simulink library "PlanarVehicle"  (R2018b)
settings: Solver=VariableStepAuto  StartTime=0.0  StopTime=10.0  RelTol=1e-3
undefined symbols (not defined in the file or in its folder): ENVIRONMENT, GEOMETRY, PROPULSION, SIMULATION
libraries: UWSimulink3DAnimationBlockset x2, UWAerospaceBlockset_FlightParameters x2, vrlib x1, UWMiscBlockset x1
settings Model: Creator=Christopher  LastModifiedBy=Christopher

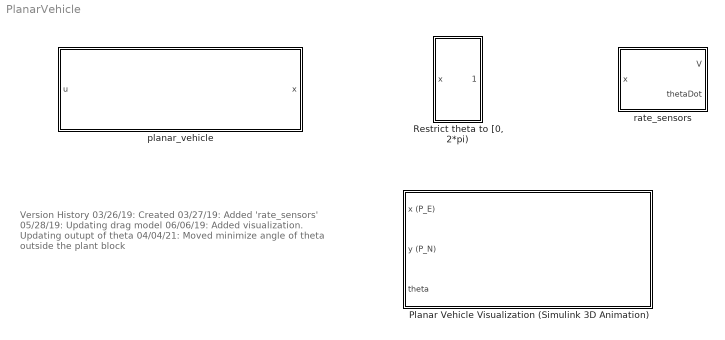
== system PlanarVehicle ==
  note: Version History
      | 03/26/19: Created
      | 03/27/19: Added 'rate_sensors'
      | 05/28/19: Updating drag model
      | 06/06/19: Added visualization.  Updating outupt of theta
      | 04/04/21: Moved minimize angle of theta outside the plant block
  Planar Vehicle Visualization (Simulink 3D Animation) : Subsystem  mask{T_animate=1}
      mask prompts: T_animate "Time step for animation"
      mask help:
      | This is a visualization of the planar vehicle using the Simulink 3D Animation environment.
      |
      | Note: Simulink should open up the VRML sink and it should display the aircraft model in a separate window.  If this does not occur, you may need to look under the mask and through down through subsystems until you find the VR Sink block.  Double click on this block to open the animation window.
      |
      | Further note that Simulink may close the VRML sink the first time it is run (it may display a warning with verbiage about 'Virtual world has been closed from outside of Simulink.'.  If this occurs, simply repeat the procedure of looking under the mask and double clicking on the VR Sink.
      |
      | INPUTS:
      | -x: x-position (position east)
      | -y: y-position (position north)
      | -theta: heading angle (0 = pointing in +y (east) direction, positive counter-clockwise) (rad)
      |
      | Christopher Lum
      | lum@uw.edu
      mask Display: image('Simulink3Visualization.png')
  "Restrict theta to [0, 2*pi)" : Subsystem
  planar_vehicle : Subsystem  mask{m=GEOMETRY.mass, Ib=GEOMETRY.Ib, Fmax=PROPULSION.Fmax, Mmax=PROPULSION.Mmax, x0=SIMULATION.X_0, CT=ENVIRONMENT.CT, CR=ENVIRONMENT.CR}
      mask prompts: m "Mass (kg)"; Ib "Moment of Inertia (kg*m^2)"; Fmax "Maximum thrust (N)"; Mmax "Maximum torque (N*m)"; x0 "Initial condition (6x1 vector)"; CT "Coefficient of translational friction (N*s^2/m^2)"; CR "Coefficient of rotational friction (N*m*s)"
      mask help:
      | Represent a simple planar model.
      |
      | The state vector is
      |
      |    x =  [x;y;xdot;ydot;theta;thetadot]
      |
      | The control vector is
      |
      |    u = [u1; u2]
      |
      | where:
      | u1 = fraction of  axial thrust force in range [-1, 1] (-1 = full nagative force, +1 = full positive force)
      | u2 = fraction of moment about CG in range [-1, 1] (-1 = full negative moment, +1 = full positive moment)
      |
      | INPUTS:
      | -u: 2x1 control vector
      |
      | OUTPUTS:
      | -x: 6x1 state vector
      |
      | For more information see PlanarVehicle.nb.
      |
      | Created by Christopher Lum
      | lum@uw.edu
      mask DialogControl Container5 Prompt: Geometry
      mask DialogControl Container9 Prompt: Propulsion
      mask DialogControl Container11 Prompt: Simulation
      mask DialogControl Container15 Prompt: Environment
      mask Display: image('Boat.png')
  rate_sensors : Subsystem
      mask help:
      | Models rate sensors which measure the translational and rotational velocity of the vehicle.
      |
      | INPUTS:
      | -x: 6x1 state vector
      |
      | OUTPUTS:
      | -V: scalar representing planar velocity (m/s)
      | -thetaDot: scalar representing rotational velocity (rad/s)
      |
      | Created by Christopher Lum
      | lum@uw.edu

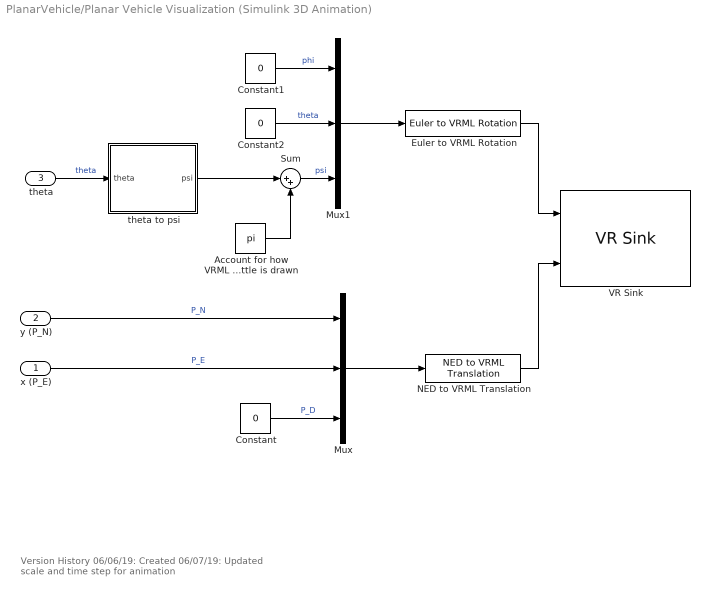
== system PlanarVehicle/Planar Vehicle Visualization (Simulink 3D Animation) ==
  note: Version History
      | 06/06/19: Created
      | 06/07/19: Updated scale and time step for animation
  x (P_E) : Inport
  y (P_N) : Inport  Port=2
  theta : Inport  Port=3
  Account for how VRML Shuttle is drawn : Constant  Value=pi
  Constant : Constant  Value=0
  Constant1 : Constant  Value=0
  Constant2 : Constant  Value=0
  Euler to VRML Rotation : UWSimulink3DAnimationBlockset/Euler to VRML Rotation
  Mux : Mux  Inputs=3
  Mux1 : Mux  Inputs=3
  NED to VRML Translation : UWSimulink3DAnimationBlockset/NED to VRML Translation
  Sum : Sum  Inputs=|++
  VR Sink : vrlib/VR Sink  InstantiateOnLoad=on  SampleTime=T_animate  ViewEnable=on  RemoteChange=off  RemoteView=off  FieldsWritten=Shuttle.rotation.4.1.1.double#Shuttle.translation.3.1.1.double  WorldFileName=PugetSound.wrl  AutoView=on  VideoDimensions=[]  AllowVariableSize=off
      settings: SourceProductBaseCode=VR
  theta to psi : Subsystem
  wires:
  Euler to VRML Rotation/1 -> VR Sink/1
  y (P_N)/1 -> Mux/1  "P_N"
  theta/1 -> theta to psi/1(theta)  "theta"
  Sum/1 -> Mux1/3  "psi"
  Constant2/1 -> Mux1/2  "theta"
  Account for how VRML Shuttle is drawn/1 -> Sum/2
  theta to psi/1(psi) -> Sum/1
  x (P_E)/1 -> Mux/2  "P_E"
  NED to VRML Translation/1 -> VR Sink/2
  Mux1/1 -> Euler to VRML Rotation/1
  Mux/1 -> NED to VRML Translation/1
  Constant/1 -> Mux/3  "P_D"
  Constant1/1 -> Mux1/1  "phi"

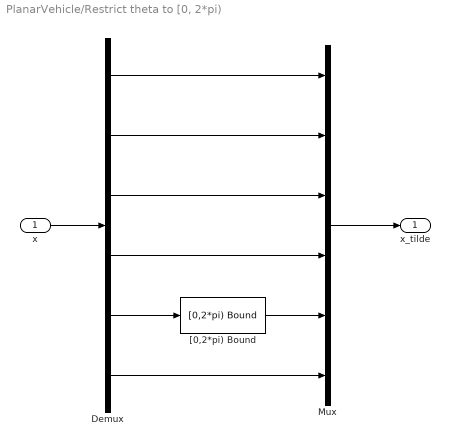
== system PlanarVehicle/Restrict theta to [0, 2*pi) ==
  "x " : Inport
  Demux : Demux  Outputs=6
  Mux : Mux  Inputs=6
  "[0,2*pi) Bound" : UWMiscBlockset/[0,2*pi) Bound  Description=|
      | Version History  
      |                  
      | 05/??/05: Created
  "  x_tilde" : Outport
  wires:
  "x "/1 -> Demux/1
  Demux/1 -> Mux/1
  Demux/2 -> Mux/2
  Demux/3 -> Mux/3
  Demux/4 -> Mux/4
  Demux/5 -> "[0,2*pi) Bound"/1
  Demux/6 -> Mux/6
  Mux/1 -> "  x_tilde"/1
  "[0,2*pi) Bound"/1 -> Mux/5

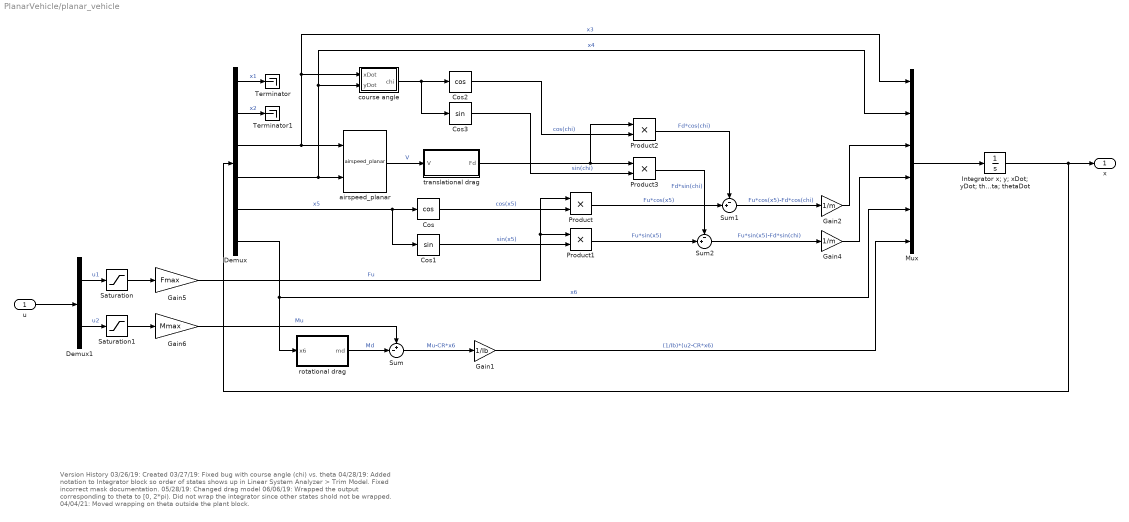
== system PlanarVehicle/planar_vehicle ==
  note: Version History
      | 03/26/19: Created
      | 03/27/19: Fixed bug with course angle (chi) vs. theta
      | 04/28/19: Added notation to Integrator block so order of states shows up in Linear System Analyzer > Trim Model.  Fixed incorrect mask documentation.
      | 05/28/19: Changed drag model
      | 06/06/19: Wrapped the output corresponding to theta to [0, 2*pi).  Did not wrap the integrator since other states shold not be wrapped.
      | 04/04/21: Moved wrapping on theta outside the plant block.
  u : Inport
  Cos : Trigonometry  Operator=cos
  Cos1 : Trigonometry
  Cos2 : Trigonometry  Operator=cos
  Cos3 : Trigonometry
  Demux : Demux  Outputs=6
  Demux1 : Demux  Outputs=2
  Gain1 : Gain  Gain=1/Ib
  Gain2 : Gain  Gain=1/m
  Gain4 : Gain  Gain=1/m
  Gain5 : Gain  Gain=Fmax
  Gain6 : Gain  Gain=Mmax
  Integrator x; y; xDot; yDot; theta; thetaDot : Integrator  InitialCondition=x0
  Mux : Mux  Inputs=6
  Product{,1..3} (4 alike) : Product
  Saturation : Saturate  UpperLimit=1  LowerLimit=-1
  Saturation1 : Saturate  UpperLimit=1  LowerLimit=-1
  Sum : Sum  Inputs=+-|
  Sum1 : Sum  Inputs=-+|
  Sum2 : Sum  Inputs=-+|
  Terminator : Terminator
  Terminator1 : Terminator
  airspeed_planar : UWAerospaceBlockset_FlightParameters/airspeed_planar
  course angle : Subsystem
  rotational drag : Subsystem
  translational drag : Subsystem
  x : Outport
  wires:
  Mux/1 -> Integrator x; y; xDot; yDot; theta; thetaDot/1
  Demux/3 -> Mux/1, course angle/1(xDot), airspeed_planar/1  "x3"
  Demux/4 -> course angle/2(yDot), Mux/2, airspeed_planar/2  "x4"
  Demux/1 -> Terminator/1  "x1"
  Demux/2 -> Terminator1/1  "x2"
  Demux/5 -> Cos1/1, Cos/1  "x5"
  Demux/6 -> rotational drag/1(x6), Mux/5  "x6"
  Sum/1 -> Gain1/1  "Mu-CR*x6"
  Gain1/1 -> Mux/6  "(1/Ib)*(u2-CR*x6)"
  Demux1/2 -> Saturation1/1  "u2"
  Cos/1 -> Product/2  "cos(x5)"
  Demux1/1 -> Saturation/1  "u1"
  Product/1 -> Sum1/2  "Fu*cos(x5)"
  Cos1/1 -> Product1/2  "sin(x5)"
  Product1/1 -> Sum2/2  "Fu*sin(x5)"
  Product2/1 -> Sum1/1  "Fd*cos(chi)"
  Product3/1 -> Sum2/1  "Fd*sin(chi)"
  Sum1/1 -> Gain2/1  "Fu*cos(x5)-Fd*cos(chi)"
  Sum2/1 -> Gain4/1  "Fu*sin(x5)-Fd*sin(chi)"
  Gain4/1 -> Mux/4
  Gain2/1 -> Mux/3
  u/1 -> Demux1/1
  course angle/1(chi) -> Cos3/1, Cos2/1
  Cos2/1 -> Product2/2  "cos(chi)"
  Cos3/1 -> Product3/2  "sin(chi)"
  Saturation/1 -> Gain5/1
  Saturation1/1 -> Gain6/1
  Gain5/1 -> Product/1, Product1/1  "Fu"
  Gain6/1 -> Sum/1  "Mu"
  rotational drag/1(md) -> Sum/2  "Md"
  translational drag/1(Fd) -> Product2/1, Product3/1
  airspeed_planar/1 -> translational drag/1(V)  "V"
  Integrator x; y; xDot; yDot; theta; thetaDot/1 -> x/1, Demux/1

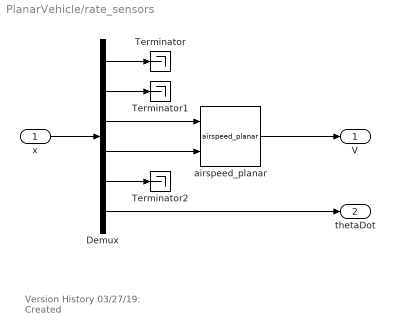
== system PlanarVehicle/rate_sensors ==
  note: Version History
      | 03/27/19: Created
  x : Inport
  Demux : Demux  Outputs=6
  Terminator : Terminator
  Terminator1 : Terminator
  Terminator2 : Terminator
  airspeed_planar : UWAerospaceBlockset_FlightParameters/airspeed_planar
  V : Outport
  thetaDot : Outport  Port=2
  wires:
  x/1 -> Demux/1
  Demux/1 -> Terminator/1
  Demux/2 -> Terminator1/1
  Demux/3 -> airspeed_planar/1
  Demux/4 -> airspeed_planar/2
  Demux/5 -> Terminator2/1
  airspeed_planar/1 -> V/1
  Demux/6 -> thetaDot/1

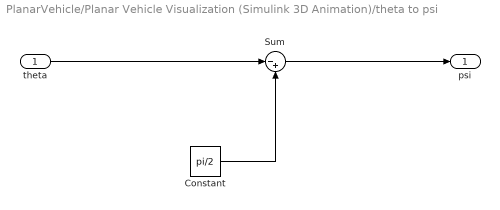
== system PlanarVehicle/Planar Vehicle Visualization (Simulink 3D Animation)/theta to psi ==
  theta : Inport
  Constant : Constant  Value=pi/2
  Sum : Sum  Inputs=|-+
  psi : Outport
  wires:
  theta/1 -> Sum/1
  Constant/1 -> Sum/2
  Sum/1 -> psi/1

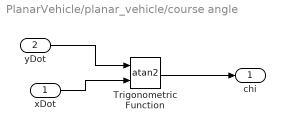
== system PlanarVehicle/planar_vehicle/course angle ==
  xDot : Inport
  yDot : Inport  Port=2
  Trigonometric Function : Trigonometry  Operator=atan2
  chi : Outport
  wires:
  yDot/1 -> Trigonometric Function/1
  xDot/1 -> Trigonometric Function/2
  Trigonometric Function/1 -> chi/1

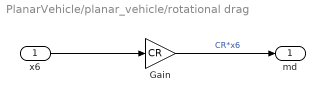
== system PlanarVehicle/planar_vehicle/rotational drag ==
  x6 : Inport
  Gain : Gain  Gain=CR
  md : Outport
  wires:
  Gain/1 -> md/1  "CR*x6"
  x6/1 -> Gain/1

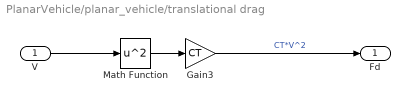
== system PlanarVehicle/planar_vehicle/translational drag ==
  V : Inport
  Gain3 : Gain  Gain=CT
  Math Function : Math  Operator=square  SaturateOnIntegerOverflow=on
  Fd : Outport
  wires:
  V/1 -> Math Function/1
  Gain3/1 -> Fd/1  "CT*V^2"
  Math Function/1 -> Gain3/1
